simulink model "DetectMIOLaneCenter"  (R2024a)
settings: configuration reference "csMultiInstance" (kept outside this file)
Description:
  | Lane Following Data Conditioning (SW Component)
settings Model: DataDictionary=DD_DetectMIOLaneCenter.sldd  EnableAccessToBaseWorkspace=off  Creator=The MathWorks, Inc.  LastModifiedBy=The MathWorks, Inc.
settings ConfigSetRef: SourceName=csMultiInstance

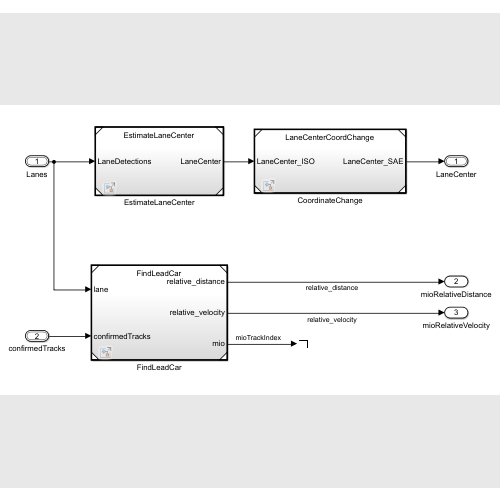
[thumbnail: Simulink's stored preview of the top-level diagram]
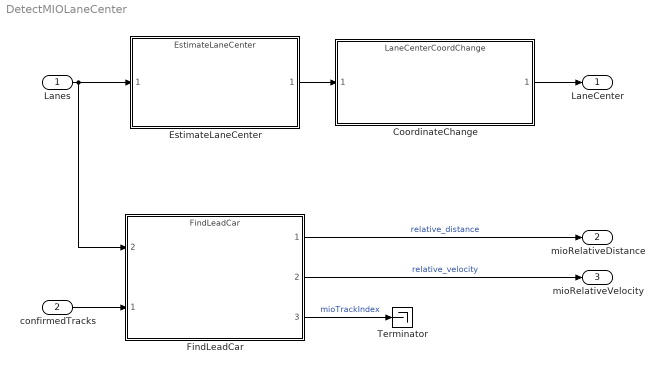
== system DetectMIOLaneCenter ==
  Lanes : Inport  OutDataTypeStr=Bus: LaneSensor
  confirmedTracks : Inport  Port=2  OutDataTypeStr=Bus: BusMultiObjectTracker  BusOutputAsStruct=on
  CoordinateChange : ModelReference  ModelNameDialog=LaneCenterCoordChange  SimulationMode=Normal  ModelReferenceVersion=8.0
  EstimateLaneCenter : ModelReference  ModelNameDialog=EstimateLaneCenter  SimulationMode=Normal  ModelReferenceVersion=8.0
  FindLeadCar : ModelReference  ModelNameDialog=FindLeadCar  SimulationMode=Normal  ModelReferenceVersion=8.0
      settings: PortSchema="{\"entries\":[{\"content\":{\"sides\":[{\"content\":{\"connectorIds\":[\"In2\",\"In1\"]},\"type\":\"ConnectorPlacement.EquallySpacedRectSide\",\"uuid\":\"4349d734-83a0-4c79-9bf4-dd7e1c5047ab\"},{\"content\":{\"connectorIds\":[\"Out1\",\"Out2\",\"Out3\"],\"side\":\"RIGHT\"},\"type\":\"ConnectorPlacement.EquallySpacedRectSide\",\"uuid\":\"3497a288-e875-428b-aa1d-01beb64c37b8\"},{\"content\":{\"connectorIds\":[],\"side\":\"TOP\"},\"type\":\"ConnectorPlacement.EquallySpacedRectSide\",\"uuid\":\"6907f1c8-6830-47d7-a2e5-b2da15eec0fd\"},{\"content\":{\"connectorIds\":[],\"side\":\"HIDDEN\"},\"type\":\"ConnectorPlacement.EquallySpacedRectSide\",\"uuid\":\"2d32d625-8302-4b7b-9dcd-25a8ceed215b\"}]},\"type\":\"ConnectorPlacement.EquallySpacedConnector\",\"uuid\":\"e7864525-b9fa-479c-8c83-c086f2216a35\"}],\"packageUris\":[\"http://schema.mathworks.com/mf0/Connector/R2020b\"],\"version\":\"1.0\"}"
  Terminator : Terminator
  LaneCenter : Outport  OutDataTypeStr=Bus: BusLaneCenter
  mioRelativeDistance : Outport  Port=2  OutDataTypeStr=double
  mioRelativeVelocity : Outport  Port=3  OutDataTypeStr=double
  wires:
  FindLeadCar/2 -> mioRelativeVelocity/1  "relative_velocity"
  FindLeadCar/1 -> mioRelativeDistance/1  "relative_distance"
  confirmedTracks/1 -> FindLeadCar/1
  Lanes/1 -> FindLeadCar/2, EstimateLaneCenter/1
  EstimateLaneCenter/1 -> CoordinateChange/1
  CoordinateChange/1 -> LaneCenter/1
  FindLeadCar/3 -> Terminator/1  "mioTrackIndex"
